simulink library "SUB_L4_Task_10ms"  (R2018a)
settings: Solver=VariableStepAuto  StartTime=0.0  StopTime=10.0  RelTol=1e-3
libraries: EmE_MBD_Blockset x75, simulink x11, SUB_L4_Task_10ms_SUB_APTC x1, SUB_L4_Task_10ms_SUB_BRKPEDARB x1, SUB_L4_Task_10ms_SUB_FAULT_MANAGER x1, SUB_L4_Task_10ms_SUB_STATE_CONTROL x1, SUB_L4_Task_10ms_SUB_STEERCTRL x1, simulink_need_slupdate x1
(part 2 of 2)

== stateflow chart SUB_L4_Task_10ms/Task_10ms/Vehicle_speed_target/Determine_sigmoid_vehicle_speed_profile/VehicleSpeedSetpointDynamicCalculation ==
  state CalculateAcceleration34 [function]
    (default) -> (junction 180) : {num = 2 * (AccelerationInitialLimited *  AccelerationFinalLimited ...
        |     - AccelerationInitialLimited * Jerk56 * TimeFinal ...
        |     + Jerk56 * (VelocityFinalLimited - VelocityInitialLimited)) ...
        |     - AccelerationInitialLimited^2 - AccelerationFinalLimited^2;
        |
        | den = 2 * ((VelocityFinalLimited - VelocityInitialLimited) ...
        |     - AccelerationFinalLimited * TimeFinal) ...
        |     + Jerk56 * TimeFinal^2;
        |
        | Jerk12 = sign(Jerk12) * max(abs(Jerk12), abs(num / den) + 0.001);
        | Jerk12 = max(-10,min(10,Jerk12));
        |
        | Calculate_abc}
    (junction 180) -> (junction 181) [order 1] : [abs(a) < 0.01 ]
    (junction 180) -> (junction 205) [order 2]
    (junction 181) -> (junction 183) : {Jerk12 = Jerk56;
        | Calculate_abc
        | Acceleration34 = - c / b;
        | AlternateMethod = false;}
    (junction 205) -> (junction 291) [order 1] : [b^2 <= 4 * a * c]
    (junction 205) -> (junction 288) [order 2] : {Acceleration34 = (- b + (b^2 - 4 * a * c)^0.5) / (2 * a);
        | AlternateMethod = false;}
    (junction 291) -> (junction 290) : {CalculateAlternate_abc
        | Acceleration34 = - b / (2 * a);
        | AlternateMethod = true;}
    (junction 290) -> (junction 288)
    (junction 183) -> (junction 290)
    (junction 288) -> (junction 189)
  state Calculate_abc [function]
    (default) -> (junction 164) : {a = Jerk56 - Jerk12;
        | b = 2 * (AccelerationFinalLimited * Jerk12 - AccelerationInitialLimited * Jerk56 - Jerk12 * Jerk56 * TimeFinal);
        | c = 2 * Jerk12 * Jerk56 * (VelocityFinalLimited - VelocityInitialLimited) + Jerk56 * AccelerationInitialLimited^2 - Jerk12 * AccelerationFinalLimited^2;}
  state CalculateAlternate_abc [function]
    (default) -> (junction 287) : {a = 1;
        | b = 2 * (Jerk56 * (TimeFinal - 0.005) - AccelerationFinalLimited);
        | c = 2 * Jerk56 * (VelocityInitialLimited - VelocityFinalLimited) + AccelerationFinalLimited^2;}
  (default) -> (junction 85)
  (junction 85) -> (junction 86) [order 1] : [Enable]
  (junction 85) -> (junction 87) [order 2]
  (junction 86) -> (junction 236) : {PositionFinalLimited = max(0.001,PositionFinal);  % limit minimum distance so that values in PositionVectorRaw are in increasing order
      |
      | VelocityInitialLimited = max(0.1,VelocityInitial);  % limit to make sure FinalTime calculation does not divide by zero
      | VelocityFinalLimited = max(0.1,VelocityFinal);  % limit to make sure FinalTime calculation does not divide by zero
      |
      | TimeFinal = 2 * PositionFinalLimited / (VelocityInitialLimited + VelocityFinalLimited);  % first approximation for total time
      | TimeFinal = max(0.007, TimeFinal);  % limit to make sure values in JerkVectorRaw are in increasing order and divide by zero protection
      |  AccelerationAverage = (VelocityFinalLimited - VelocityInitialLimited) / TimeFinal;   % acceleration with straight line velocity change
      | TimeFinal = 2 * TimeFinal;  % increase initial estimate two times to make sure solution is within search range
      | }
  (junction 236) -> (junction 237) [order 1] : [VelocityFinalLimited > VelocityInitialLimited]
  (junction 236) -> (junction 38) [order 2] : {% deceleration sigmoid limits
      | AccelerationInitialLimited = max(AccelerationAverage, min(0, AccelerationInitial));
      | AccelerationFinalLimited = max(AccelerationAverage, min(0, AccelerationFinal));}
  (junction 237) -> (junction 239) : {% acceleration sigmoid limits
      | AccelerationInitialLimited = max(0, min(AccelerationAverage, AccelerationInitial));
      | AccelerationFinalLimited = max(0, min(AccelerationAverage, AccelerationFinal));}
  (junction 239) -> (junction 38)
  (junction 38) -> (junction 21) : {DeltaTimeFinal = TimeFinal;  % initialize DeltaTimeFinal term for binary search
      | i = 1;}
  (junction 21) -> (junction 19) [order 1] : % TimeFinal
      | % Binary Search
      |
      | [i <= 15]
  (junction 19) -> (junction 115) : {JerkFinalMinimum = 2 * (VelocityInitialLimited - VelocityFinalLimited + AccelerationFinalLimited * TimeFinal) / TimeFinal^2;}
  (junction 115) -> (junction 117) [order 1] : [VelocityFinalLimited > VelocityInitialLimited]
  (junction 115) -> (junction 269) [order 2] : {% deceleration
      | Jerk12 = -JerkMagnitudeInitial;
      | Jerk56 = max(abs(JerkFinalMinimum), JerkMagnitudeFinal);}
  (junction 117) -> (junction 119) : {% acceleration
      | Jerk12 = JerkMagnitudeInitial;
      | Jerk56 = -max(abs(JerkFinalMinimum), JerkMagnitudeFinal);}
  (junction 119) -> (junction 269)
  (junction 269) -> (junction 25) : {CalculateAcceleration34}
  (junction 25) -> (junction 143) [order 1] : [abs(Acceleration34 - AccelerationAverage) < 0.001]
  (junction 25) -> (junction 297) [order 2]
  (junction 143) -> (junction 149) : {Time12 = 0.002;
      | Time56 = 0.002;
      |
      | TimeVectorRaw = [0; Time12 - 0.001; Time12 + 0.001; ...
      |     TimeFinal - Time56 - 0.001; TimeFinal - Time56 + 0.001;TimeFinal];
      |
      | JerkVectorRaw = [0; 0; 0; 0; 0; 0];
      | AccelerationVectorRaw(1) = AccelerationAverage;}
  (junction 297) -> (junction 299) [order 1] : [AlternateMethod]
  (junction 297) -> (junction 156) [order 2] : {Time12 = max(0.002, (Acceleration34 - AccelerationInitialLimited) / Jerk12);
      | Time56 = max(0.002, (AccelerationFinalLimited - Acceleration34) / Jerk56);
      |
      | TimeVectorRaw = [0; Time12 - 0.001; Time12 + 0.001; ...
      |     TimeFinal - Time56 - 0.001; TimeFinal - Time56 + 0.001;TimeFinal];
      |
      | JerkVectorRaw = [Jerk12; Jerk12; 0; 0; Jerk56; Jerk56];
      | AccelerationVectorRaw(1) = AccelerationInitialLimited;}
  (junction 299) -> (junction 301) : {Time12 = 0.002;
      | Time56 = max(0.002, (AccelerationFinalLimited - Acceleration34) / Jerk56);
      |
      | TimeVectorRaw = [0; Time12 - 0.001; Time12 + 0.001; ...
      |     TimeFinal - Time56 - 0.001; TimeFinal - Time56 + 0.001;TimeFinal];
      |
      | JerkVectorRaw = [0; 0; 0; 0; Jerk56; Jerk56];
      | AccelerationVectorRaw(1) = Acceleration34;}
  (junction 301) -> (junction 156)
  (junction 149) -> (junction 301)
  (junction 22) -> (junction 21) : {i = i + 1;}
  (junction 21) -> (junction 23) [order 2]
  (junction 156) -> (junction 32) : {VelocityVectorRaw(1) = VelocityInitialLimited;
      | PositionVectorRaw(1) = 0;
      | j = 2;}
  (junction 32) -> (junction 35) [order 1] : [j <= 6]
  (junction 35) -> (junction 31) : {DeltaTime = TimeVectorRaw(j) - TimeVectorRaw(j-1);
      | AverageJerk = 0.5 * (JerkVectorRaw(j-1) + JerkVectorRaw(j));
      | AccelerationVectorRaw(j) = AccelerationVectorRaw(j-1) + JerkVectorRaw(j-1) * DeltaTime;
      | VelocityVectorRaw(j) = VelocityVectorRaw(j-1) + AccelerationVectorRaw(j-1) * DeltaTime + 0.5 * JerkVectorRaw(j-1) * DeltaTime^2;
      | PositionVectorRaw(j) = PositionVectorRaw(j-1) + VelocityVectorRaw(j-1) * DeltaTime + 0.5 * AccelerationVectorRaw(j-1) * DeltaTime^2 + (JerkVectorRaw(j-1) / 6) * DeltaTime^3;}
  (junction 31) -> (junction 32) : {j = j + 1;}
  (junction 32) -> (junction 56) [order 2] : {PositionError = PositionVectorRaw(end) - PositionFinalLimited;
      | DeltaTimeFinal = 0.5 * DeltaTimeFinal;  % reduce DeltaTimeFinal by 50 percent on each iteration of the search
      | }
  (junction 56) -> (junction 57) [order 1] : [(PositionError < 0) && (VelocityVectorRaw(end) > 0)]
  (junction 56) -> (junction 59) [order 2] : {TimeFinal = TimeFinal - DeltaTimeFinal;}
  (junction 57) -> (junction 58) : {TimeFinal = TimeFinal + DeltaTimeFinal;}
  (junction 58) -> (junction 59)
  (junction 59) -> (junction 22) : {TimeFinal = max(0.007, TimeFinal);}
  (junction 23) -> (junction 87)
  (junction 87) -> (junction 92)
  data: TimeVectorRaw output size=6 =[0:0.001:0.005]'; PositionVectorRaw output size=6 =[0:0.001:0.005]'; VelocityVectorRaw output size=6 =zeros(6,1); AccelerationVectorRaw output size=6 =zeros(6,1); JerkVectorRaw output size=6 =zeros(6,1); Enable input boolean; PositionFinal input; VelocityInitial input; VelocityFinal input; AccelerationInitial input; AccelerationFinal input; TimeFinal local double; AccelerationAverage local double; DeltaTimeFinal local double; i local uint8; j local uint8; DeltaTime local double; AverageJerk local double; PositionError local double; JerkError local double; PositionFinalLimited local double; VelocityInitialLimited local double; VelocityFinalLimited local double; AccelerationInitialLimited local double; AccelerationFinalLimited local double; Jerk56 local double; Jerk12 local double; JerkMagnitudeInitial input; JerkMagnitudeFinal input; a local double; b local double; c local double; Acceleration34 local double; Time12 local double; Time56 local double; JerkFinalMinimum local double; AlternateMethod local boolean; num local double; den local double
